simulink model "Generic_13"  (R2022b)
settings: Solver=VariableStepAuto  StartTime=0.0  StopTime=10.0  RelTol=1e-3
values from neighbouring files (symbols this model uses):
  A = cell2mat(A_cell)    [MPCController1.m]    (also in MPC_Fmincon.m)
  B = cell2mat(B_cell)    [MPCController1.m]    (also in MPC_Fmincon.m)
  brake_select = ones(length(speed), length(steering_angle))    [TwoDLook_uptable.m]
  curvature = 0.000:0.001:1    [TwoDLook_uptable.m]
  m = 1600    [MPCController1.m]    (also in MPCController2.m; MPC_Fmincon.m)
  speed = 0:0.1:100    [TwoDLook_uptable.m]
undefined symbols (not defined in the file or in its folder): Amplifier, DiscIntNeverNeededParam, K_d_yawrate, K_dsteering, k_speed, k_stanley, kd, ki, kp, path_curvature
libraries: CarMaker4SL x121, simulink x12, cstblocks x7, autolibshared x1, mpcadaslib x1
(part 2 of 5)

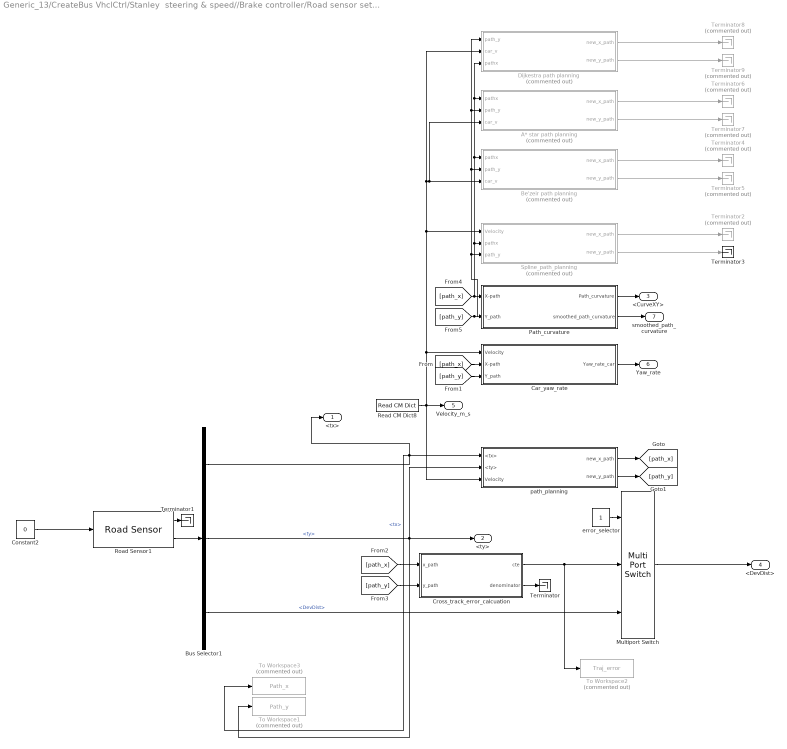
== system Generic_13/CreateBus VhclCtrl/Stanley  steering & speed//Brake controller/Road sensor set & path planning/Road sensor set & path planning ==
  A* star path planning : Subsystem  Commented=on
  Be'zeir path planning : Subsystem  Commented=on
  Bus Selector1 : BusSelector  OutputSignals=Path.tx,Path.ty,Path.DevDist
  Car_yaw_rate : Subsystem
  Constant2 : Constant  Value=0
  Cross_track_error_calcuation : Subsystem
  Dijkestra path planning : Subsystem  Commented=on
  Multiport Switch : MultiPortSwitch  Inputs=2  SaturateOnIntegerOverflow=off  InputSameDT=off
  Path_curvature : Subsystem
  Read CM Dict8 : CarMaker4SL/Read CM Dict  xname=Vhcl.v  xsync=off  xstime=Continuous
  Road Sensor1 : CarMaker4SL/Sensors/Road Sensor  xname=0  xstime=Continuous
      settings: SourceProductName=CarMaker4SL
  Spline_path_planning : Subsystem  Commented=on
  Terminator : Terminator
  Terminator1 : Terminator
  Terminator{2,4..9} (7 alike) : Terminator  Commented=on
  Terminator3 : Terminator
  To Workspace1 : ToWorkspace  Commented=on  VariableName=Path_y  SampleTime=-1
      settings: Save2DSignal=2-D array (concatenate along first dimension)
  To Workspace2 : ToWorkspace  Commented=on  VariableName=Traj_error  SampleTime=-1
      settings: Save2DSignal=2-D array (concatenate along first dimension)
  To Workspace3 : ToWorkspace  Commented=on  VariableName=Path_x  SampleTime=-1
      settings: Save2DSignal=2-D array (concatenate along first dimension)
  error_selector : Constant
  path_planning : Subsystem
  <tx> : Outport
  <ty> : Outport  Port=2
  <CurveXY> : Outport  Port=3
  <DevDist> : Outport  Port=4
  Velocity_m_s : Outport  Port=5
  Yaw_rate : Outport  Port=6
  smoothed_path_curvature : Outport  Port=7
  wires:
  [path_x] -> Car_yaw_rate/2(X-path)
  [path_x] -> Cross_track_error_calcuation/1(x_path)
  Bus Selector1/2 -> path_planning/2(<ty>), To Workspace1/1, <ty>/1  "<ty>"
  Road Sensor1/2 -> Bus Selector1/1
  Constant2/1 -> Road Sensor1/1
  Path_curvature/1(Path_curvature) -> <CurveXY>/1
  Road Sensor1/1 -> Terminator1/1
  [path_y] -> Cross_track_error_calcuation/2(y_path)
  [path_y] -> Car_yaw_rate/3(Y_path)
  Bus Selector1/1 -> path_planning/1(<tx>), To Workspace3/1, <tx>/1  "<tx>"
  Bus Selector1/3 -> Multiport Switch/3  "<DevDist>"
  error_selector/1 -> Multiport Switch/1
  Cross_track_error_calcuation/1(cte) -> To Workspace2/1, Multiport Switch/2
  Cross_track_error_calcuation/2(denominator) -> Terminator/1
  Car_yaw_rate/1(Yaw_rate_car) -> Yaw_rate/1
  path_planning/1(new_x_path) -> [path_x]
  path_planning/2(new_y_path) -> [path_y]
  Multiport Switch/1 -> <DevDist>/1
  Path_curvature/2(smoothed_path_curvature) -> smoothed_path_curvature/1
  Spline_path_planning/2(new_y_path) -> Terminator3/1
  Spline_path_planning/1(new_x_path) -> Terminator2/1
  Be'zeir path planning/1(new_x_path) -> Terminator4/1
  Be'zeir path planning/2(new_y_path) -> Terminator5/1
  [path_y] -> Dijkestra path planning/1(path_y), A* star path planning/2(path_y), Be'zeir path planning/2(path_y), Spline_path_planning/3(path_y), Path_curvature/2(Y_path)
  [path_x] -> Dijkestra path planning/3(pathx), A* star path planning/1(pathx), Be'zeir path planning/1(pathx), Spline_path_planning/2(pathx), Path_curvature/1(X-path)
  A* star path planning/2(new_y_path) -> Terminator7/1
  A* star path planning/1(new_x_path) -> Terminator6/1
  Dijkestra path planning/1(new_x_path) -> Terminator8/1
  Dijkestra path planning/2(new_y_path) -> Terminator9/1
  Read CM Dict8/1 -> Velocity_m_s/1, Dijkestra path planning/2(car_v), A* star path planning/3(car_v), Be'zeir path planning/3(car_v), Spline_path_planning/1(Velocity), Car_yaw_rate/1(Velocity), path_planning/3(Velocity)

== system Generic_13/CreateBus VhclCtrl/Stanley  steering & speed//Brake controller/Stanley controller with path_planning/Stanley controller with path_planning ==
  X-path : Inport
  Y_path : Inport  Port=2
  Discrete-Time Integrator1 : DiscreteIntegrator  Commented=on  SampleTime=-1  ICPrevOutput=DiscIntNeverNeededParam  ICPrevScaledInput=DiscIntNeverNeededParam
  MATLAB Function : MATLAB Function  Commented=on  TreatAsAtomicUnit=on
  MATLAB Function1 : MATLAB Function  Commented=on  TreatAsAtomicUnit=on
  Path_Calculation_V02 : MATLAB Function  Commented=on  TreatAsAtomicUnit=on
  Read CM Dict10 : CarMaker4SL/Read CM Dict  Commented=on  xname=Vhcl.v  xsync=off  xstime=Continuous
  Read CM Dict11 : CarMaker4SL/Read CM Dict  Commented=on  xname=Car.Gen.tx  xsync=off  xstime=Continuous
  Read CM Dict13 : CarMaker4SL/Read CM Dict  Commented=on  xname=Car.YawRate  xsync=off  xstime=Continuous
  Read CM Dict7 : CarMaker4SL/Read CM Dict  Commented=on  xname=Car.Road.Path.DevDist  xsync=off  xstime=Continuous
  Read CM Dict9 : CarMaker4SL/Read CM Dict  Commented=on  xname=Car.Gen.ty  xsync=off  xstime=Continuous
  Saturation : Saturate  Commented=on  UpperLimit=1.6  LowerLimit=-1.6
  Subsystem3 : Subsystem  Commented=on
  X_Global_Pos_m : Subsystem  Commented=on
  Y_Global_Pos_m : Subsystem  Commented=on
  Yaw_angle_rad : Subsystem  Commented=on
  e : Outport
  err_fr_axle : Outport  Port=2
  cross_track_steering : Outport  Port=3
  heading_err : Outport  Port=4
  Steering : Outport  Port=5
  closest_point : Outport  Port=6
  wires:
  X-path/1 -> Subsystem3/1(X-path)
  MATLAB Function/5(steering) -> Saturation/1
  X_Global_Pos_m/1(Pos_X) -> MATLAB Function1/1(Pos_X)
  Y_path/1 -> Subsystem3/2(Y_path)
  Subsystem3/1(x_path) -> Path_Calculation_V02/3(path_x)
  Read CM Dict13/1 -> Discrete-Time Integrator1/1, MATLAB Function/3(yaw)
  Read CM Dict9/1 -> Y_Global_Pos_m/1(In1), Path_Calculation_V02/2(y_car)
  Read CM Dict11/1 -> X_Global_Pos_m/1(In1), Path_Calculation_V02/1(x_car)
  Subsystem3/2(y_path) -> Path_Calculation_V02/4(y_path)
  Discrete-Time Integrator1/1 -> Yaw_angle_rad/1(In1)
  Y_Global_Pos_m/1(Pos_Y) -> MATLAB Function1/2(Pos_Y)
  Path_Calculation_V02/1(closest_point) -> closest_point/1
  Path_Calculation_V02/2(instantaneous_path) -> MATLAB Function1/4(Path_In)
  Yaw_angle_rad/1(Yaw_Angle) -> MATLAB Function1/3(Yaw_Angle)
  MATLAB Function1/1(Path_Out) -> MATLAB Function/1(path)
  Read CM Dict7/1 -> MATLAB Function/2(dev)
  Read CM Dict10/1 -> MATLAB Function/4(speed_act)
  MATLAB Function/1(e) -> e/1
  MATLAB Function/2(err_fr_axle) -> err_fr_axle/1
  MATLAB Function/3(cross_track_steering) -> cross_track_steering/1
  MATLAB Function/4(heading_err) -> heading_err/1
  Saturation/1 -> Steering/1  "Steering"

== system Generic_13/CreateBus VhclCtrl/Stanley  steering & speed//Brake controller/Stanley_controller_vfin/Stanley_controller_vfin ==
  Velocity : Inport
  Curvature : Inport  Port=2
  Vehicle_yaw_rate : Inport  Port=3
  Path.DevDist : Inport  Port=4
  Stanley_standfort controller : Subsystem  VariantControl=Choice
  Steering angle : Outport
  dev_angle : Outport  Port=2

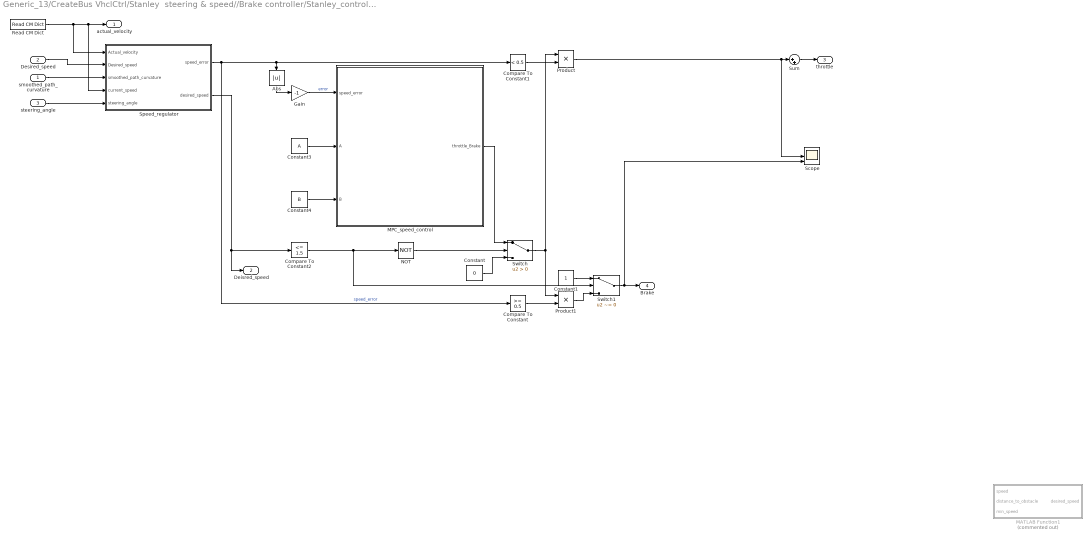
== system Generic_13/CreateBus VhclCtrl/Stanley  steering & speed//Brake controller/Stanley_controller_with_thottle_and_brake_commands/MPCLongitudianl_contorl ==
  smoothed_path_curvature : Inport
  Desired_speed : Inport  Port=2
  steering_angle : Inport  Port=3
  Abs : Abs  SaturateOnIntegerOverflow=off
  Compare To Constant : simulink/Logic and Bit Operations/Compare To Constant  relop=>=  const=0.5  OutDataTypeStr=boolean
  Compare To Constant1 : simulink/Logic and Bit Operations/Compare To Constant  relop=<  const=0.5  OutDataTypeStr=boolean
  Compare To Constant2 : simulink/Logic and Bit Operations/Compare To Constant  relop=<=  const=1.5  OutDataTypeStr=boolean
  Constant : Constant  Value=0
  Constant1 : Constant
  Constant3 : Constant  Value=A
  Constant4 : Constant  Value=B
  Gain : Gain  Gain=-1
  MATLAB Function1 : MATLAB Function  Commented=on  TreatAsAtomicUnit=on
  MPC_speed_control : MATLAB Function  TreatAsAtomicUnit=on
  NOT : Logic  Operator=NOT  IconShape=distinctive  AllPortsSameDT=off  OutDataTypeStr=boolean
  Product : Product
  Product1 : Product
  Read CM Dict : CarMaker4SL/Read CM Dict  xname=Vhcl.v  xsync=off  xstime=Continuous
  Scope : Scope  NumInputPorts=3
  Speed_regulator : Subsystem
  Sum : Sum  Inputs=|++
  Switch : Switch  Criteria=u2 > Threshold  SaturateOnIntegerOverflow=off  InputSameDT=off
  Switch1 : Switch  Criteria=u2 ~= 0  SaturateOnIntegerOverflow=off  InputSameDT=off
  actual_velocity : Outport
  Deisred_speed : Outport  Port=2
  throttle : Outport  Port=3
  Brake : Outport  Port=4
  wires:
  Read CM Dict/1 -> Speed_regulator/4(current_speed), actual_velocity/1, Speed_regulator/1(Actual_velocity)
  Abs/1 -> Gain/1
  Speed_regulator/2(desired_speed) -> Compare To Constant2/1, Deisred_speed/1
  steering_angle/1 -> Speed_regulator/5(steering_angle)
  Speed_regulator/1(speed_error) -> Compare To Constant1/1, Abs/1, Compare To Constant/1  "speed_error"
  Desired_speed/1 -> Speed_regulator/2(Desired_speed)
  smoothed_path_curvature/1 -> Speed_regulator/3(smoothed_path_curvature)
  Gain/1 -> MPC_speed_control/1(speed_error)  "error"
  Constant4/1 -> MPC_speed_control/3(B)
  Constant3/1 -> MPC_speed_control/2(A)
  Compare To Constant2/1 -> Switch1/2, NOT/1
  NOT/1 -> Switch/2
  Constant/1 -> Switch/3
  Compare To Constant1/1 -> Product/2
  Switch/1 -> Product/1, Product1/1
  Compare To Constant/1 -> Product1/2
  Product/1 -> Scope/2, Sum/1
  Constant1/1 -> Switch1/1
  Product1/1 -> Switch1/3
  Switch1/1 -> Scope/3, Brake/1
  MPC_speed_control/1(throttle_Brake) -> Switch/1
  Sum/1 -> throttle/1

== system Generic_13/CreateBus VhclCtrl/Stanley  steering & speed//Brake controller/Stanley_controller_with_thottle_and_brake_commands/Stanley steering + PID speed controller ==
  Path_out : Inport
  <Vx_Global_m_s> : Inport  Port=2
  <Vy_Global_m_s> : Inport  Port=3
  dev_angle : Inport  Port=4
  <Actual_Velocity_Car_m_s> : Inport  Port=5
  Desired_speed : Inport  Port=6
  dev_distance : Inport  Port=7
  Actual velocity [km/h] : Display
  Bus Selector : BusSelector  OutputSignals=Path.tx,Path.ty
  Constant1 : Constant  Value=0
  Delay : Delay  DelayLength=1
  Delay1 : Delay  DelayLength=1
  Gain : Gain  Gain=3.6
  Road Sensor : CarMaker4SL/Sensors/Road Sensor  xname=0  xstime=Continuous
      settings: SourceProductName=CarMaker4SL
  Saturation : Saturate  UpperLimit=pi()/2  LowerLimit=-pi/2
  Smoothing : Subsystem
  Speed_controller : Subsystem
  Stanely_controller : MATLAB Function  TreatAsAtomicUnit=on
  Subsystem1 : Subsystem
  Terminator : Terminator
  Terminator1 : Terminator
  Terminator4 : Terminator
  Steering_angle_rad : Outport  VectorParamsAs1DForOutWhenUnconnected=off
  Throttle : Outport  Port=2
  Brake_command : Outport  Port=3
  wires:
  dev_distance/1 -> Stanely_controller/2(dev)  "Dev_dis[m]"
  <Vx_Global_m_s>/1 -> Speed_controller/3(velocity_x)
  Constant1/1 -> Road Sensor/1
  dev_angle/1 -> Stanely_controller/1(dev_angle)  "dev_angle [rad]"
  <Vy_Global_m_s>/1 -> Speed_controller/4(velocity_y)
  Bus Selector/2 -> Stanely_controller/6(y2), Delay1/1  "<ty>"
  Speed_controller/4(min_safe_speed) -> Subsystem1/3(min_safe_speed)
  Road Sensor/1 -> Terminator4/1
  Road Sensor/2 -> Bus Selector/1
  Bus Selector/1 -> Stanely_controller/4(x2), Delay/1  "<tx>"
  Delay/1 -> Stanely_controller/3(x1)
  Delay1/1 -> Stanely_controller/5(y1)
  <Actual_Velocity_Car_m_s>/1 -> Speed_controller/2(speed_act), Gain/1, Stanely_controller/7(speed_act)
  Desired_speed/1 -> Subsystem1/1(desired_speed)
  Speed_controller/2(Brake_command) -> Brake_command/1
  Stanely_controller/3(steering) -> Speed_controller/6(steering), Saturation/1  "steering"
  Gain/1 -> Actual velocity [km/h]/1  "Actual velocity [km/h]"
  Path_out/1 -> Speed_controller/1(path)
  Subsystem1/1(Target_speed) -> Speed_controller/5(desired_speed)
  Saturation/1 -> Smoothing/1(Signal_In)  "Control signal"
  Speed_controller/1(Throttle) -> Throttle/1
  Speed_controller/3(path_curvature) -> Subsystem1/2(curvature)
  Smoothing/1(Signal_Out) -> Steering_angle_rad/1
  Stanely_controller/2(cross_track_steering) -> Terminator/1  "cross_track_steering"
  Stanely_controller/1(e) -> Terminator1/1  "cross track error [m]"

== system Generic_13/CreateBus VhclCtrl/Stanley  steering & speed//Brake controller/Road sensor set & path planning/Road sensor set & path planning/A* star path planning ==
  pathx : Inport
  path_y : Inport  Port=2
  car_v : Inport  Port=3
  Basic_obstacle avoidance : MATLAB Function  TreatAsAtomicUnit=on
  Demux : Demux  Commented=on
  Discrete-Time Integrator : DiscreteIntegrator  SampleTime=-1  ICPrevOutput=DiscIntNeverNeededParam  ICPrevScaledInput=DiscIntNeverNeededParam
  Mux : Mux  Inputs=2
  Mux1 : Mux  Inputs=2
  Read CM Dict : CarMaker4SL/Read CM Dict  xname=Sensor.Object.RadarL.Obj.T00.RefPnt.ds.x  xsync=off  xstime=Continuous
  Read CM Dict1 : CarMaker4SL/Read CM Dict  xname=Sensor.Object.RadarL.Obj.T00.RefPnt.ds.y  xsync=off  xstime=Continuous
  Read CM Dict2 : CarMaker4SL/Read CM Dict  xname=Car.Gen.tx  xsync=off  xstime=Continuous
  Read CM Dict3 : CarMaker4SL/Read CM Dict  xname=Car.Gen.ty  xsync=off  xstime=Continuous
  Read CM Dict4 : CarMaker4SL/Read CM Dict  xname=Sensor.Radar.VehSensor_6.Obj0.Width  xsync=off  xstime=Continuous
  Read CM Dict5 : CarMaker4SL/Read CM Dict  xname=Sensor.Radar.VehSensor_6.Obj0.Length  xsync=off  xstime=Continuous
  Read CM Dict6 : CarMaker4SL/Read CM Dict  xname=Car.YawRate  xsync=off  xstime=Continuous
  Reshape : Reshape  OutputDimensionality=Customize  OutputDimensions=[2,1]
  Reshape1 : Reshape  OutputDimensionality=Customize  OutputDimensions=[1,2]
  Reshape4 : Reshape  Commented=on
  Saturation : Saturate  UpperLimit=4  LowerLimit=-4
  Signal_smoothing : Subsystem
  Smoothing3 : Subsystem
  getInstantaneousPath Function : MATLAB Function  Commented=on  TreatAsAtomicUnit=on
  lookahead_dist : Constant  Commented=on  Value=2
  new_x_path : Outport
  new_y_path : Outport  Port=2
  wires:
  Reshape4/1 -> Demux/1
  Demux/4 -> new_y_path/1
  Basic_obstacle avoidance/1(updated_path) -> getInstantaneousPath Function/1(generated_path), Reshape4/1
  Demux/1 -> new_x_path/1
  lookahead_dist/1 -> getInstantaneousPath Function/2(lookahead_distance)
  pathx/1 -> Basic_obstacle avoidance/8(path_x), Mux1/1
  path_y/1 -> Basic_obstacle avoidance/9(path_y), Mux1/2
  car_v/1 -> Basic_obstacle avoidance/7(car_v)
  Smoothing3/1(Signal_Out) -> Basic_obstacle avoidance/5(object_length)  "steering_signal"
  Signal_smoothing/1(smoothed_width) -> Basic_obstacle avoidance/6(object_width)
  Saturation/1 -> Smoothing3/1(Signal_In)
  Discrete-Time Integrator/1 -> getInstantaneousPath Function/4(current_heading)
  Reshape/1 -> getInstantaneousPath Function/3(current_position)
  Mux1/1 -> Reshape1/1
  Read CM Dict5/1 -> Saturation/1
  Read CM Dict6/1 -> Discrete-Time Integrator/1
  Mux/1 -> Reshape/1
  Read CM Dict3/1 -> Basic_obstacle avoidance/2(Car_y), Mux/2
  Read CM Dict4/1 -> Signal_smoothing/1(Signal_In)
  Read CM Dict2/1 -> Basic_obstacle avoidance/1(Car_x), Mux/1
  Read CM Dict1/1 -> Basic_obstacle avoidance/4(dy)
  Read CM Dict/1 -> Basic_obstacle avoidance/3(dx)

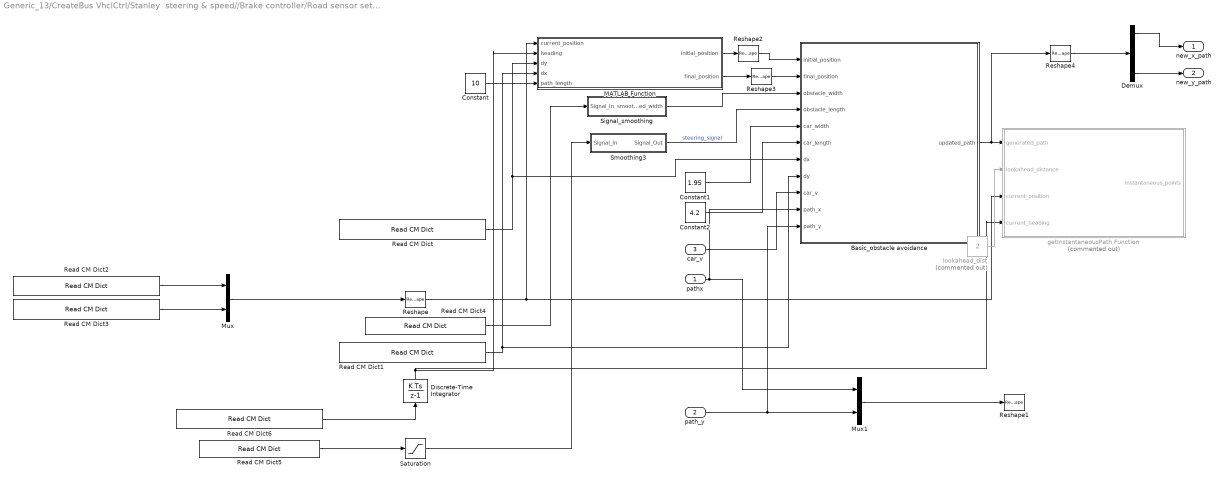
== system Generic_13/CreateBus VhclCtrl/Stanley  steering & speed//Brake controller/Road sensor set & path planning/Road sensor set & path planning/Be'zeir path planning ==
  pathx : Inport
  path_y : Inport  Port=2
  car_v : Inport  Port=3
  Basic_obstacle avoidance : MATLAB Function  TreatAsAtomicUnit=on
  Constant : Constant  Value=10
  Constant1 : Constant  Value=1.95
  Constant2 : Constant  Value=4.2
  Demux : Demux
  Discrete-Time Integrator : DiscreteIntegrator  SampleTime=-1  ICPrevOutput=DiscIntNeverNeededParam  ICPrevScaledInput=DiscIntNeverNeededParam
  MATLAB Function : MATLAB Function  TreatAsAtomicUnit=on
  Mux : Mux  Inputs=2
  Mux1 : Mux  Inputs=2
  Read CM Dict : CarMaker4SL/Read CM Dict  xname=Sensor.Object.RadarL.Obj.T00.RefPnt.ds.x  xsync=off  xstime=Continuous
  Read CM Dict1 : CarMaker4SL/Read CM Dict  xname=Sensor.Object.RadarL.Obj.T00.RefPnt.ds.y  xsync=off  xstime=Continuous
  Read CM Dict2 : CarMaker4SL/Read CM Dict  xname=Car.Gen.tx  xsync=off  xstime=Continuous
  Read CM Dict3 : CarMaker4SL/Read CM Dict  xname=Car.Gen.ty  xsync=off  xstime=Continuous
  Read CM Dict4 : CarMaker4SL/Read CM Dict  xname=Sensor.Radar.VehSensor_6.Obj0.Width  xsync=off  xstime=Continuous
  Read CM Dict5 : CarMaker4SL/Read CM Dict  xname=Sensor.Radar.VehSensor_6.Obj0.Length  xsync=off  xstime=Continuous
  Read CM Dict6 : CarMaker4SL/Read CM Dict  xname=Car.YawRate  xsync=off  xstime=Continuous
  Reshape : Reshape  OutputDimensionality=Customize  OutputDimensions=[2,1]
  Reshape1 : Reshape  OutputDimensionality=Customize  OutputDimensions=[1,2]
  Reshape2 : Reshape  OutputDimensionality=Customize  OutputDimensions=[1,2]
  Reshape3 : Reshape  OutputDimensionality=Customize  OutputDimensions=[1,2]
  Reshape4 : Reshape
  Saturation : Saturate  UpperLimit=4  LowerLimit=-4
  Signal_smoothing : Subsystem
  Smoothing3 : Subsystem
  getInstantaneousPath Function : MATLAB Function  Commented=on  TreatAsAtomicUnit=on
  lookahead_dist : Constant  Commented=on  Value=2
  new_x_path : Outport
  new_y_path : Outport  Port=2
  wires:
  Read CM Dict1/1 -> Basic_obstacle avoidance/8(dy), MATLAB Function/4(dx)
  Read CM Dict2/1 -> Mux/1
  MATLAB Function/2(final_position) -> Reshape3/1
  Constant/1 -> MATLAB Function/5(path_length)
  Read CM Dict4/1 -> Signal_smoothing/1(Signal_In)
  Read CM Dict3/1 -> Mux/2
  Mux/1 -> Reshape/1
  Read CM Dict6/1 -> Discrete-Time Integrator/1
  Read CM Dict5/1 -> Saturation/1
  Mux1/1 -> Reshape1/1
  Read CM Dict/1 -> Basic_obstacle avoidance/7(dx), MATLAB Function/3(dy)
  Reshape/1 -> getInstantaneousPath Function/3(current_position), MATLAB Function/1(current_position)
  Discrete-Time Integrator/1 -> MATLAB Function/2(heading), getInstantaneousPath Function/4(current_heading)
  Saturation/1 -> Smoothing3/1(Signal_In)
  MATLAB Function/1(initial_position) -> Reshape2/1
  Signal_smoothing/1(smoothed_width) -> Basic_obstacle avoidance/3(obstacle_width)
  Constant1/1 -> Basic_obstacle avoidance/5(car_width)
  Smoothing3/1(Signal_Out) -> Basic_obstacle avoidance/4(obstacle_length)  "steering_signal"
  Constant2/1 -> Basic_obstacle avoidance/6(car_length)
  car_v/1 -> Basic_obstacle avoidance/9(car_v)
  path_y/1 -> Mux1/2, Basic_obstacle avoidance/11(path_y)
  pathx/1 -> Mux1/1, Basic_obstacle avoidance/10(path_x)
  lookahead_dist/1 -> getInstantaneousPath Function/2(lookahead_distance)
  Reshape2/1 -> Basic_obstacle avoidance/1(initial_position)
  Reshape3/1 -> Basic_obstacle avoidance/2(final_position)
  Demux/1 -> new_x_path/1
  Basic_obstacle avoidance/1(updated_path) -> Reshape4/1, getInstantaneousPath Function/1(generated_path)
  Demux/4 -> new_y_path/1
  Reshape4/1 -> Demux/1

== system Generic_13/CreateBus VhclCtrl/Stanley  steering & speed//Brake controller/Road sensor set & path planning/Road sensor set & path planning/Car_yaw_rate ==
  Velocity : Inport
  X-path : Inport  Port=2
  Y_path : Inport  Port=3
  " Path_expanding1" : Subsystem
  Constant : Constant  Value=20
  Gain2 : Gain  Gain=-1
  Multiport Switch : MultiPortSwitch  Inputs=2  SaturateOnIntegerOverflow=off  InputSameDT=off
  Multiport Switch1 : MultiPortSwitch  Inputs=2  SaturateOnIntegerOverflow=off  InputSameDT=off
  Product3 : Product
  Read CM Dict5 : CarMaker4SL/Read CM Dict  xname=Car.YawRate  xsync=off  xstime=Continuous
  Saturation3 : Saturate  UpperLimit=5  LowerLimit=-5
  Varying Lowpass Filter1 : cstblocks/Linear Parameter Varying/Varying Lowpass Filter  N=1
  Vehicle_yaw_rate_selcotr : Constant
  Yaw_rate_filter_slector : Constant
  calculate_path_curvature2 : MATLAB Function  TreatAsAtomicUnit=on  VariantControl=Choice
  Yaw_rate_car : Outport
  wires:
  " Path_expanding1"/1(x_path) -> calculate_path_curvature2/1(path_x)
  X-path/1 -> " Path_expanding1"/1(X-path)
  Gain2/1 -> Multiport Switch1/2, Saturation3/1
  Y_path/1 -> " Path_expanding1"/2(Y_path)
  Velocity/1 -> Product3/1
  " Path_expanding1"/2(y_path) -> calculate_path_curvature2/2(path_y)
  Product3/1 -> Gain2/1
  calculate_path_curvature2/1(path_curvature) -> Product3/2
  Saturation3/1 -> Varying Lowpass Filter1/1
  Constant/1 -> Varying Lowpass Filter1/2
  Yaw_rate_filter_slector/1 -> Multiport Switch1/1
  Varying Lowpass Filter1/1 -> Multiport Switch1/3  "Yaw_rate_car"
  Vehicle_yaw_rate_selcotr/1 -> Multiport Switch/1
  Multiport Switch1/1 -> Multiport Switch/2
  Read CM Dict5/1 -> Multiport Switch/3
  Multiport Switch/1 -> Yaw_rate_car/1  "Yaw_rate_car"

== system Generic_13/CreateBus VhclCtrl/Stanley  steering & speed//Brake controller/Road sensor set & path planning/Road sensor set & path planning/Cross_track_error_calcuation ==
  x_path : Inport
  y_path : Inport  Port=2
  Constant : Constant  Value=25
  Cross_track_error_calcuation : MATLAB Function  TreatAsAtomicUnit=on
  Delay : Delay  DelayLength=1  InitialCondition=0.1
  Delay1 : Delay  DelayLength=1  InitialCondition=0.1
  Gain1 : Gain  Gain=-1
  Read CM Dict12 : CarMaker4SL/Read CM Dict  xname=Car.Gen.ty  xsync=off  xstime=Continuous
  Read CM Dict8 : CarMaker4SL/Read CM Dict  xname=Car.Gen.tx  xsync=off  xstime=Continuous
  Saturation1 : Saturate  UpperLimit=7  LowerLimit=-7
  Varying Lowpass Filter2 : cstblocks/Linear Parameter Varying/Varying Lowpass Filter  N=1
  cte : Outport
  denominator : Outport  Port=2
  wires:
  Read CM Dict12/1 -> Cross_track_error_calcuation/2(y_vehicle)
  x_path/1 -> Cross_track_error_calcuation/5(x2), Delay1/1
  Saturation1/1 -> Varying Lowpass Filter2/1
  Delay/1 -> Cross_track_error_calcuation/4(y_point)
  Cross_track_error_calcuation/2(denominator) -> denominator/1
  y_path/1 -> Cross_track_error_calcuation/6(y2), Delay/1
  Delay1/1 -> Cross_track_error_calcuation/3(x_point)
  Read CM Dict8/1 -> Cross_track_error_calcuation/1(x_vehicle)
  Cross_track_error_calcuation/1(cte) -> Gain1/1
  Gain1/1 -> Saturation1/1
  Constant/1 -> Varying Lowpass Filter2/2
  Varying Lowpass Filter2/1 -> cte/1

== system Generic_13/CreateBus VhclCtrl/Stanley  steering & speed//Brake controller/Road sensor set & path planning/Road sensor set & path planning/Dijkestra path planning ==
  path_y : Inport
  car_v : Inport  Port=2
  pathx : Inport  Port=3
  Basic_obstacle avoidance : MATLAB Function  TreatAsAtomicUnit=on
  Demux : Demux  Commented=on
  Discrete-Time Integrator : DiscreteIntegrator  SampleTime=-1  ICPrevOutput=DiscIntNeverNeededParam  ICPrevScaledInput=DiscIntNeverNeededParam
  Mux : Mux  Inputs=2
  Mux1 : Mux  Inputs=2
  Read CM Dict : CarMaker4SL/Read CM Dict  xname=Sensor.Object.RadarL.Obj.T00.RefPnt.ds.x  xsync=off  xstime=Continuous
  Read CM Dict1 : CarMaker4SL/Read CM Dict  xname=Sensor.Object.RadarL.Obj.T00.RefPnt.ds.y  xsync=off  xstime=Continuous
  Read CM Dict2 : CarMaker4SL/Read CM Dict  xname=Car.Gen.tx  xsync=off  xstime=Continuous
  Read CM Dict3 : CarMaker4SL/Read CM Dict  xname=Car.Gen.ty  xsync=off  xstime=Continuous
  Read CM Dict4 : CarMaker4SL/Read CM Dict  xname=Sensor.Radar.VehSensor_6.Obj0.Width  xsync=off  xstime=Continuous
  Read CM Dict5 : CarMaker4SL/Read CM Dict  xname=Sensor.Radar.VehSensor_6.Obj0.Length  xsync=off  xstime=Continuous
  Read CM Dict6 : CarMaker4SL/Read CM Dict  xname=Car.YawRate  xsync=off  xstime=Continuous
  Reshape : Reshape  OutputDimensionality=Customize  OutputDimensions=[2,1]
  Reshape1 : Reshape  OutputDimensionality=Customize  OutputDimensions=[1,2]
  Reshape4 : Reshape  Commented=on
  Saturation : Saturate  UpperLimit=4  LowerLimit=-4
  Signal_smoothing : Subsystem
  Smoothing3 : Subsystem
  getInstantaneousPath Function : MATLAB Function  Commented=on  TreatAsAtomicUnit=on
  lookahead_dist : Constant  Commented=on  Value=2
  new_x_path : Outport
  new_y_path : Outport  Port=2
  wires:
  Read CM Dict/1 -> Basic_obstacle avoidance/3(dx)
  Read CM Dict1/1 -> Basic_obstacle avoidance/4(dy)
  Read CM Dict2/1 -> Mux/1, Basic_obstacle avoidance/1(Car_x)
  Read CM Dict4/1 -> Signal_smoothing/1(Signal_In)
  Read CM Dict3/1 -> Mux/2, Basic_obstacle avoidance/2(Car_y)
  Mux/1 -> Reshape/1
  Read CM Dict6/1 -> Discrete-Time Integrator/1
  Read CM Dict5/1 -> Saturation/1
  Mux1/1 -> Reshape1/1
  Reshape/1 -> getInstantaneousPath Function/3(current_position)
  Discrete-Time Integrator/1 -> getInstantaneousPath Function/4(current_heading)
  Saturation/1 -> Smoothing3/1(Signal_In)
  Signal_smoothing/1(smoothed_width) -> Basic_obstacle avoidance/6(object_width)
  Smoothing3/1(Signal_Out) -> Basic_obstacle avoidance/5(object_length)  "steering_signal"
  car_v/1 -> Basic_obstacle avoidance/7(car_v)
  path_y/1 -> Mux1/2, Basic_obstacle avoidance/9(path_y)
  pathx/1 -> Mux1/1, Basic_obstacle avoidance/8(path_x)
  lookahead_dist/1 -> getInstantaneousPath Function/2(lookahead_distance)
  Demux/1 -> new_x_path/1
  Basic_obstacle avoidance/1(updated_path) -> Reshape4/1, getInstantaneousPath Function/1(generated_path)
  Demux/4 -> new_y_path/1
  Reshape4/1 -> Demux/1

== system Generic_13/CreateBus VhclCtrl/Stanley  steering & speed//Brake controller/Road sensor set & path planning/Road sensor set & path planning/Path_curvature ==
  X-path : Inport
  Y_path : Inport  Port=2
  " Path_expanding" : Subsystem
  Constant : Constant  Value=25
  Multiport Switch : MultiPortSwitch  Inputs=2  SaturateOnIntegerOverflow=off  InputSameDT=off
  Multiport Switch1 : MultiPortSwitch  Inputs=2  SaturateOnIntegerOverflow=off  InputSameDT=off
  Read CM Dict6 : CarMaker4SL/Read CM Dict  xname=Sensor.Road.VehSensor_0.Path.CurveXY  xsync=off  xstime=Continuous
  Saturation2 : Saturate  UpperLimit=1  LowerLimit=-1
  Scope : Scope
  Varying Lowpass Filter : cstblocks/Linear Parameter Varying/Varying Lowpass Filter  N=1
  calculate_path_curvature1 : MATLAB Function  TreatAsAtomicUnit=on  VariantControl=Choice
  inverting : Gain  Gain=-1
  path_curv_selector : Constant
  path_curv_selector1 : Constant
  Path_curvature : Outport
  smoothed_path_curvature : Outport  Port=2
  wires:
  inverting/1 -> Multiport Switch1/2, Saturation2/1
  X-path/1 -> " Path_expanding"/1(X-path)
  Y_path/1 -> " Path_expanding"/2(Y_path)
  " Path_expanding"/1(x_path) -> calculate_path_curvature1/1(path_x)
  calculate_path_curvature1/1(path_curvature) -> inverting/1
  Read CM Dict6/1 -> Multiport Switch/3
  " Path_expanding"/2(y_path) -> calculate_path_curvature1/2(path_y)
  Saturation2/1 -> Varying Lowpass Filter/1
  Varying Lowpass Filter/1 -> Scope/1, smoothed_path_curvature/1, Multiport Switch1/3  "Path_curvature"
  Constant/1 -> Varying Lowpass Filter/2
  path_curv_selector1/1 -> Multiport Switch1/1
  path_curv_selector/1 -> Multiport Switch/1
  Multiport Switch1/1 -> Multiport Switch/2
  Multiport Switch/1 -> Path_curvature/1  "Path_curvature"

== system Generic_13/CreateBus VhclCtrl/Stanley  steering & speed//Brake controller/Road sensor set & path planning/Road sensor set & path planning/Spline_path_planning ==
  Velocity : Inport
  pathx : Inport  Port=2
  path_y : Inport  Port=3
  Demux : Demux  Outputs=2
  Discrete-Time Integrator : DiscreteIntegrator  SampleTime=-1  ICPrevOutput=DiscIntNeverNeededParam  ICPrevScaledInput=DiscIntNeverNeededParam
  Mux : Mux  Inputs=2
  Mux1 : Mux  Inputs=2
  Read CM Dict : CarMaker4SL/Read CM Dict  xname=Sensor.Object.RadarL.Obj.T00.RefPnt.ds.x  xsync=off  xstime=Continuous
  Read CM Dict1 : CarMaker4SL/Read CM Dict  xname=Sensor.Object.RadarL.Obj.T00.RefPnt.ds.y  xsync=off  xstime=Continuous
  Read CM Dict2 : CarMaker4SL/Read CM Dict  xname=Car.Gen.tx  xsync=off  xstime=Continuous
  Read CM Dict3 : CarMaker4SL/Read CM Dict  xname=Car.Gen.ty  xsync=off  xstime=Continuous
  Read CM Dict4 : CarMaker4SL/Read CM Dict  xname=Sensor.Radar.VehSensor_6.Obj0.Width  xsync=off  xstime=Continuous
  Read CM Dict5 : CarMaker4SL/Read CM Dict  xname=Sensor.Radar.VehSensor_6.Obj0.Length  xsync=off  xstime=Continuous
  Read CM Dict6 : CarMaker4SL/Read CM Dict  xname=Car.YawRate  xsync=off  xstime=Continuous
  Reshape : Reshape  OutputDimensionality=Customize  OutputDimensions=[1,2]
  Reshape1 : Reshape  OutputDimensionality=Customize  OutputDimensions=[1,2]
  Saturation : Saturate  UpperLimit=4  LowerLimit=-4
  Signal_smoothing : Subsystem
  Smoothing3 : Subsystem
  Spline_bsed_obstacle avoidance : MATLAB Function  TreatAsAtomicUnit=on
  getInstantaneousPath Function : MATLAB Function  TreatAsAtomicUnit=on
  lookahead_dist : Constant  Value=2
  new_x_path : Outport
  new_y_path : Outport  Port=2
  wires:
  Signal_smoothing/1(smoothed_width) -> Spline_bsed_obstacle avoidance/5(object_width)
  Read CM Dict4/1 -> Signal_smoothing/1(Signal_In)
  Demux/1 -> new_x_path/1
  Demux/2 -> new_y_path/1
  Spline_bsed_obstacle avoidance/1(updated_path) -> getInstantaneousPath Function/1(generated_path)  "generated_path"
  Smoothing3/1(Signal_Out) -> Spline_bsed_obstacle avoidance/6(object_length)  "steering_signal"
  Read CM Dict1/1 -> Spline_bsed_obstacle avoidance/4(dy)
  Read CM Dict/1 -> Spline_bsed_obstacle avoidance/3(dx)
  Saturation/1 -> Smoothing3/1(Signal_In)
  Velocity/1 -> Spline_bsed_obstacle avoidance/7(car_v)
  Read CM Dict5/1 -> Saturation/1
  Read CM Dict3/1 -> Mux/2, Spline_bsed_obstacle avoidance/2(Car_y)  "car_y"
  Read CM Dict2/1 -> Mux/1, Spline_bsed_obstacle avoidance/1(Car_x)  "car_x"
  Mux/1 -> Reshape/1
  Reshape/1 -> getInstantaneousPath Function/3(current_position)
  lookahead_dist/1 -> getInstantaneousPath Function/2(lookahead_distance)
  Read CM Dict6/1 -> Discrete-Time Integrator/1
  Discrete-Time Integrator/1 -> getInstantaneousPath Function/4(current_heading)
  Mux1/1 -> Reshape1/1
  pathx/1 -> Spline_bsed_obstacle avoidance/8(pathx), Mux1/1
  path_y/1 -> Spline_bsed_obstacle avoidance/9(path_y), Mux1/2
  getInstantaneousPath Function/1(instantaneous_points) -> Demux/1

== system Generic_13/CreateBus VhclCtrl/Stanley  steering & speed//Brake controller/Road sensor set & path planning/Road sensor set & path planning/path_planning ==
  <tx> : Inport
  <ty> : Inport  Port=2
  Velocity : Inport  Port=3
  Basic_obstacle avoidance : MATLAB Function  TreatAsAtomicUnit=on
  Demux : Demux  Outputs=2
  Floor : Rounding  Operator=ceil
  Read CM Dict : CarMaker4SL/Read CM Dict  xname=Sensor.Object.FrontRadar.Obj.T00.RefPnt.ds.x  xsync=off  xstime=Continuous
  Read CM Dict1 : CarMaker4SL/Read CM Dict  xname=Sensor.Object.FrontRadar.Obj.T00.RefPnt.ds.y  xsync=off  xstime=Continuous
  Read CM Dict2 : CarMaker4SL/Read CM Dict  xname=Car.Gen.tx  xsync=off  xstime=Continuous
  Read CM Dict3 : CarMaker4SL/Read CM Dict  xname=Car.Gen.ty  xsync=off  xstime=Continuous
  Read CM Dict4 : CarMaker4SL/Read CM Dict  xname=Sensor.Radar.VehSensor_6.Obj0.Width  xsync=off  xstime=Continuous
  Read CM Dict5 : CarMaker4SL/Read CM Dict  xname=Sensor.Radar.VehSensor_6.Obj0.Length  xsync=off  xstime=Continuous
  Saturation : Saturate  UpperLimit=4  LowerLimit=-4
  Signal_smoothing : Subsystem
  Smoothing3 : Subsystem
  To Workspace1 : ToWorkspace  VariableName=CarY  SampleTime=-1
      settings: Save2DSignal=2-D array (concatenate along first dimension)
  To Workspace3 : ToWorkspace  VariableName=CarX  SampleTime=-1
      settings: Save2DSignal=2-D array (concatenate along first dimension)
  new_x_path : Outport
  new_y_path : Outport  Port=2
  wires:
  Read CM Dict2/1 -> To Workspace3/1, Basic_obstacle avoidance/1(Car_x)
  Read CM Dict3/1 -> To Workspace1/1, Basic_obstacle avoidance/2(Car_y)
  Read CM Dict5/1 -> Saturation/1
  Velocity/1 -> Basic_obstacle avoidance/9(car_v), Floor/1
  Saturation/1 -> Smoothing3/1(Signal_In)
  Read CM Dict/1 -> Basic_obstacle avoidance/3(dx)
  Read CM Dict1/1 -> Basic_obstacle avoidance/4(dy)
  Smoothing3/1(Signal_Out) -> Basic_obstacle avoidance/6(object_length)  "steering_signal"
  <tx>/1 -> Basic_obstacle avoidance/7(path_x)
  <ty>/1 -> Basic_obstacle avoidance/8(path_y)
  Floor/1 -> Basic_obstacle avoidance/10(car_v_ceil)
  Basic_obstacle avoidance/1(updated_path) -> Demux/1
  Demux/2 -> new_y_path/1
  Demux/1 -> new_x_path/1
  Read CM Dict4/1 -> Signal_smoothing/1(Signal_In)
  Signal_smoothing/1(smoothed_width) -> Basic_obstacle avoidance/5(object_width)

== system Generic_13/CreateBus VhclCtrl/Stanley  steering & speed//Brake controller/Stanley controller with path_planning/Stanley controller with path_planning/Subsystem3 ==
  X-path : Inport
  Y_path : Inport  Port=2
  Delay37 : Delay  DelayLength=1
  Delay4 : Delay  DelayLength=1
  Mux1 : Mux  Inputs=2
  Mux2 : Mux  Inputs=2
  Reshape1 : Reshape  OutputDimensionality=Customize  OutputDimensions=[1,2]
  Reshape2 : Reshape  OutputDimensionality=Customize  OutputDimensions=[1,2]
  x_path : Outport
  y_path : Outport  Port=2
  wires:
  X-path/1 -> Delay37/1, Mux2/1
  Y_path/1 -> Delay4/1, Mux1/1
  Delay37/1 -> Mux2/2
  Mux1/1 -> Reshape1/1
  Reshape1/1 -> y_path/1
  Delay4/1 -> Mux1/2
  Reshape2/1 -> x_path/1
  Mux2/1 -> Reshape2/1

== system Generic_13/CreateBus VhclCtrl/Stanley  steering & speed//Brake controller/Stanley controller with path_planning/Stanley controller with path_planning/X_Global_Pos_m ==
  In1 : Inport
  Pos_X : Outport  VectorParamsAs1DForOutWhenUnconnected=off
  wires:
  In1/1 -> Pos_X/1

== system Generic_13/CreateBus VhclCtrl/Stanley  steering & speed//Brake controller/Stanley controller with path_planning/Stanley controller with path_planning/Y_Global_Pos_m ==
  In1 : Inport
  Pos_Y : Outport  VectorParamsAs1DForOutWhenUnconnected=off
  wires:
  In1/1 -> Pos_Y/1

== system Generic_13/CreateBus VhclCtrl/Stanley  steering & speed//Brake controller/Stanley controller with path_planning/Stanley controller with path_planning/Yaw_angle_rad ==
  In1 : Inport
  Yaw_Angle : Outport  VectorParamsAs1DForOutWhenUnconnected=off
  wires:
  In1/1 -> Yaw_Angle/1

== system Generic_13/CreateBus VhclCtrl/Stanley  steering & speed//Brake controller/Stanley_controller_vfin/Stanley_controller_vfin/Stanley_standfort controller ==
  note: Vehicle_paramters
  note: Parameters
  note: K_dsteering = 10;
  note: Amplifier = -5.94
  note: K_d_yawrate =0.4
  note: Vehicle overall mass [kg] 	: 	1600.00
      |
      |  Vehicle overall center of gravity x / y / z [m] 	: 	2.596	0.000	0.562
      |
      |  Vehicle overall inertia tensor [kgm²] 	: 	696.215	0.000	-8.863
      |  	 									0.000	2707.206	0.000
      |  	 									-8.863	0.000	2986.624
  note: Distance CoG to front axle / rear axle [m] : 1.488 -1.487
  note: k_stanly = 13.6;
  Velocity : Inport
  Curvature : Inport  Port=2
  Vehicle_yaw_rate : Inport  Port=3
  Path.DevDist : Inport  Port=4
  Add : Sum  Inputs=+++
  Add1 : Sum
  Crosstrack_steering : Subsystem
  Deviation_angle_calc : Subsystem
  Scope : Scope  NumInputPorts=2
  Steady_state_yaw : Subsystem  Commented=on
  Steering_correction_facotr : Subsystem
  Yaw_rate_diff : Subsystem
  Steering angle : Outport
  dev_angle : Outport  Port=2
  wires:
  Velocity/1 -> Crosstrack_steering/1(speed), Deviation_angle_calc/1(Velocity), Yaw_rate_diff/1(Velocity)
  Crosstrack_steering/1(Cross_track_steering) -> Add/1  "Crosstrack_steering"
  Add/1 -> Add1/1
  Add1/1 -> Steering angle/1, Steering_correction_facotr/1(Steering_i+1), Steering_correction_facotr/2(Steering_i)  "Steering angle"
  Deviation_angle_calc/1(Dev_angle) -> dev_angle/1, Add/3
  Steering_correction_facotr/1(Factor_of_correction) -> Add1/2
  Yaw_rate_diff/1(Yaw_rate_factor) -> Add/2
  Vehicle_yaw_rate/1 -> Yaw_rate_diff/3(Car_yaw_rate), Deviation_angle_calc/3(Car.YawRate), Scope/2
  Path.DevDist/1 -> Crosstrack_steering/2(Path.DevDist)
  Curvature/1 -> Scope/1, Deviation_angle_calc/2(Curvature), Yaw_rate_diff/2(Curvature)

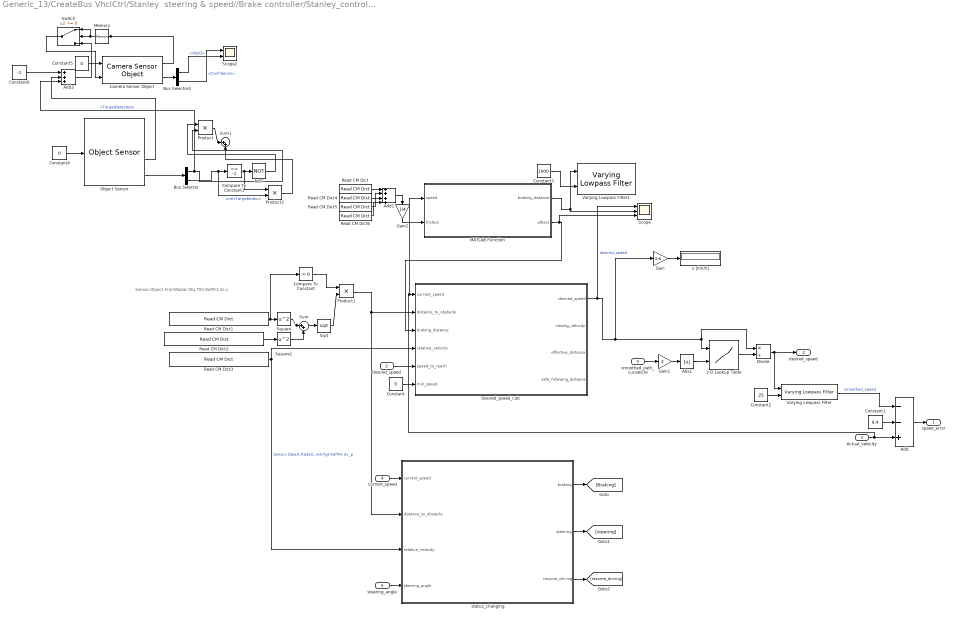
== system Generic_13/CreateBus VhclCtrl/Stanley  steering & speed//Brake controller/Stanley_controller_with_thottle_and_brake_commands/MPCLongitudianl_contorl/Speed_regulator ==
  note: Sensor.Object.FrontRadar.Obj.T00.RefPnt.ds.x
  Actual_velocity : Inport
  Desired_speed : Inport  Port=2
  smoothed_path_curvature : Inport  Port=3
  current_speed : Inport  Port=4
  steering_angle : Inport  Port=5
  2-D Lookup Table : Lookup_n-D  BreakpointsForDimension1=speed  BreakpointsForDimension2=curvature  Table=brake_select  InternalRulePriority=Speed  RndMeth=Simplest
      settings: InputPortMap=u0,u1
  Abs2 : Abs  SaturateOnIntegerOverflow=off
  Add : Sum  Inputs=--+
  Add1 : Sum  Inputs=++++
  Add2 : Sum  Inputs=+++
  Bus Selector : BusSelector  OutputSignals=TargetDetected,relvTargetIndex
  Bus Selector4 : BusSelector  OutputSignals=ObjID,Confidence
  Camera Sensor Object : CarMaker4SL/Sensors/Camera Sensor Object  xname=INPORT  xstime=Continuous
      settings: SourceProductName=CarMaker4SL
  Compare To Constant : simulink/Logic and Bit Operations/Compare To Constant  relop=>  const=0  OutDataTypeStr=boolean
  Compare To Constant1 : simulink/Logic and Bit Operations/Compare To Constant  relop===  const=-1  OutDataTypeStr=boolean
  Constant : Constant  Value=0
  Constant1 : Constant  Value=0.4
  Constant2 : Constant  Value=25
  Constant3 : Constant  Value=1000
  Constant4 : Constant  Value=0
  Constant5 : Constant  Value=0
  Constant6 : Constant  Value=-1
  Desired_speed_calc : MATLAB Function  TreatAsAtomicUnit=on
  Divide : Product  Inputs=*/
  Gain : Gain  Gain=3.6
  Gain1 : Gain  Gain=2
  Gain2 : Gain  Gain=1/4
  MATLAB Function : MATLAB Function  TreatAsAtomicUnit=on
  Memory : Memory
  NOT : Logic  Operator=NOT  IconShape=distinctive  AllPortsSameDT=off  OutDataTypeStr=boolean
  Object Sensor : CarMaker4SL/Sensors/Object Sensor  xname=INPORT  xstime=Continuous
      settings: SourceProductName=CarMaker4SL
  Product : Product
  Product1 : Product
  Product2 : Product
  Read CM Dict : CarMaker4SL/Read CM Dict  xname=Car.muRoadFL  xsync=off  xstime=Continuous
  Read CM Dict1 : CarMaker4SL/Read CM Dict  xname=Sensor.Object.FrontRadar.Obj.T01.RefPnt.ds.x  xsync=off  xstime=Continuous
  Read CM Dict2 : CarMaker4SL/Read CM Dict  xname=Sensor.Object.FrontRadar.Obj.T01.RefPnt.ds.y  xsync=off  xstime=Continuous
  Read CM Dict3 : CarMaker4SL/Read CM Dict  xname=Sensor.Object.FrontRadar.relvTgt.RefPnt.dv_p  xsync=off  xstime=Continuous
  Read CM Dict4 : CarMaker4SL/Read CM Dict  xname=Car.muRoadFR  xsync=off  xstime=Continuous
  Read CM Dict5 : CarMaker4SL/Read CM Dict  xname=Car.muRoadRL  xsync=off  xstime=Continuous
  Read CM Dict6 : CarMaker4SL/Read CM Dict  xname=Car.muRoadRR  xsync=off  xstime=Continuous
  Scope : Scope  NumInputPorts=3
  Scope2 : Scope  NumInputPorts=2
  Sqrt : Sqrt
  Square : Math  Operator=square
  Square1 : Math  Operator=square
  Sum : Sum  Inputs=|++
  Sum1 : Sum  Inputs=|++
  Switch : Switch  SaturateOnIntegerOverflow=off  InputSameDT=off
  Varying Lowpass Filter : cstblocks/Linear Parameter Varying/Varying Lowpass Filter  N=1
  Varying Lowpass Filter1 : cstblocks/Linear Parameter Varying/Varying Lowpass Filter  N=1
  status_changing : MATLAB Function  TreatAsAtomicUnit=on
  v [km/h] : Display
  speed_error : Outport
  desired_speed : Outport  Port=2
  wires:
  Gain1/1 -> Abs2/1
  Constant/1 -> Desired_speed_calc/6(min_speed)
  Sqrt/1 -> Product1/2
  Desired_speed/1 -> Desired_speed_calc/5(speed_to_reach)
  Abs2/1 -> 2-D Lookup Table/2
  Read CM Dict3/1 -> status_changing/3(relative_velocity), Desired_speed_calc/4(relative_velocity)  "Sensor.Object.RadarL.relvTgt.RefPnt.dv_p"
  Constant1/1 -> Add/2
  Product1/1 -> status_changing/2(distance_to_obstacle), Desired_speed_calc/2(distance_to_obstacle)
  Desired_speed_calc/1(desired_speed) -> Scope/1, Gain/1, Divide/1, 2-D Lookup Table/1  "desired_speed"
  Read CM Dict2/1 -> Square1/1
  steering_angle/1 -> status_changing/4(steering_angle)
  Square1/1 -> Sum/2
  Gain/1 -> v [km/h]/1
  2-D Lookup Table/1 -> Divide/2
  status_changing/3(resume_driving) -> [resume_driving]
  Sum/1 -> Sqrt/1
  Square/1 -> Sum/1
  Add/1 -> speed_error/1
  smoothed_path_curvature/1 -> Gain1/1
  Compare To Constant/1 -> Product1/1
  Read CM Dict1/1 -> Compare To Constant/1, Square/1
  status_changing/2(steering) -> [steering]
  status_changing/1(braking) -> [Braking]
  current_speed/1 -> status_changing/1(current_speed)
  Constant2/1 -> Varying Lowpass Filter/2
  Divide/1 -> desired_speed/1, Varying Lowpass Filter/1
  Varying Lowpass Filter/1 -> Add/1  "smoothed_speed"
  Actual_velocity/1 -> MATLAB Function/1(speed), Desired_speed_calc/1(current_speed), Add/3
  MATLAB Function/1(braking_distance) -> Varying Lowpass Filter1/1, Scope/2
  Constant3/1 -> Varying Lowpass Filter1/2
  Read CM Dict/1 -> Add1/1
  Read CM Dict4/1 -> Add1/2
  Read CM Dict5/1 -> Add1/3
  Read CM Dict6/1 -> Add1/4
  Add1/1 -> Gain2/1
  MATLAB Function/2(others) -> Scope/3, Desired_speed_calc/3(braking_distance)
  Gain2/1 -> MATLAB Function/2(friction)
  Object Sensor/3 -> Add2/2
  Constant4/1 -> Object Sensor/1
  Object Sensor/4 -> Bus Selector/1
  Bus Selector/2 -> Product2/2, Compare To Constant1/1  "<relvTargetIndex>"
  Compare To Constant1/1 -> Product2/1, NOT/1
  NOT/1 -> Product/1
  Product2/1 -> Sum1/2
  Bus Selector/1 -> Add2/3, Product/2  "<TargetDetected>"
  Product/1 -> Sum1/1
  Camera Sensor Object/2 -> Bus Selector4/1
  Bus Selector4/1 -> Scope2/2  "<ObjID>"
  Constant5/1 -> Camera Sensor Object/1
  Bus Selector4/2 -> Scope2/1  "<Confidence>"
  Add2/1 -> Switch/3
  Constant6/1 -> Add2/1
  Camera Sensor Object/1 -> Memory/1
  Switch/1 -> Camera Sensor Object/2
  Memory/1 -> Switch/1, Switch/2

== system Generic_13/CreateBus VhclCtrl/Stanley  steering & speed//Brake controller/Stanley_controller_with_thottle_and_brake_commands/Stanley steering + PID speed controller/Smoothing ==
  Signal_In : Inport
  Add : Sum  Inputs=++++
  Delay : Delay  InitialCondition=0.1
  Delay1 : Delay  DelayLength=4  InitialCondition=0.1
  Delay2 : Delay  DelayLength=5  InitialCondition=0.1
  Gain : Gain  Gain=0.35
  Gain1 : Gain  Gain=0.25
  Gain2 : Gain  Gain=0.25
  Gain3 : Gain  Gain=0.15
  Signal_Out : Outport  VectorParamsAs1DForOutWhenUnconnected=off
  wires:
  Gain1/1 -> Add/2
  Signal_In/1 -> Gain/1
  Delay/1 -> Gain1/1
  Gain/1 -> Add/1
  Delay1/1 -> Gain2/1
  Add/1 -> Delay2/1, Delay1/1, Delay/1, Signal_Out/1
  Gain2/1 -> Add/3
  Delay2/1 -> Gain3/1
  Gain3/1 -> Add/4

== system Generic_13/CreateBus VhclCtrl/Stanley  steering & speed//Brake controller/Stanley_controller_with_thottle_and_brake_commands/Stanley steering + PID speed controller/Speed_controller ==
  path : Inport
  speed_act : Inport  Port=2
  velocity_x : Inport  Port=3
  velocity_y : Inport  Port=4
  desired_speed : Inport  Port=5
  steering : Inport  Port=6
  Brake Saturation : Saturate  UpperLimit=1  LowerLimit=0
  Constant1 : Constant  Value=kd
  Constant2 : Constant  Value=ki
  Constant3 : Constant  Value=kp
  Path_curvature : Constant  Value=path_curvature
  Scaling factor : Gain  Gain=1/1000
  Scalling factor : Gain  Gain=1/1000
  Throttle Saturation : Saturate  UpperLimit=1  LowerLimit=-1
  advancedPID_speed_and_brake_control : MATLAB Function  TreatAsAtomicUnit=on
  calculate_path_curvature : MATLAB Function  TreatAsAtomicUnit=on
  Throttle : Outport
  Brake_command : Outport  Port=2
  path_curvature : Outport  Port=3
  min_safe_speed : Outport  Port=4
  wires:
  advancedPID_speed_and_brake_control/1(throttle) -> Scaling factor/1  "throttle"
  path/1 -> calculate_path_curvature/1(path)
  speed_act/1 -> advancedPID_speed_and_brake_control/3(speed_act)
  calculate_path_curvature/2(min_safe_speed) -> min_safe_speed/1, advancedPID_speed_and_brake_control/2(min_s_speed)  "min_s_speed"
  velocity_y/1 -> calculate_path_curvature/2(velocity_y)
  velocity_x/1 -> calculate_path_curvature/3(velocity_x)
  steering/1 -> calculate_path_curvature/4(steering_angel)
  calculate_path_curvature/1(path_curvature) -> path_curvature/1
  Constant3/1 -> advancedPID_speed_and_brake_control/7(Kp_speed)
  Path_curvature/1 -> advancedPID_speed_and_brake_control/1(path_curv)
  desired_speed/1 -> advancedPID_speed_and_brake_control/4(desired_speed)
  Constant2/1 -> advancedPID_speed_and_brake_control/6(Ki_speed)
  Constant1/1 -> advancedPID_speed_and_brake_control/5(Kd_speed)
  advancedPID_speed_and_brake_control/2(brake_cmd) -> Scalling factor/1  "Brake cmd"
  Scaling factor/1 -> Throttle Saturation/1
  Throttle Saturation/1 -> Throttle/1  "Throttle_command"
  Scalling factor/1 -> Brake Saturation/1
  Brake Saturation/1 -> Brake_command/1  "Brake_command"

== system Generic_13/CreateBus VhclCtrl/Stanley  steering & speed//Brake controller/Stanley_controller_with_thottle_and_brake_commands/Stanley steering + PID speed controller/Subsystem1 ==
  desired_speed : Inport
  curvature : Inport  Port=2
  min_safe_speed : Inport  Port=3
  2-D Lookup Table : Lookup_n-D  BreakpointsForDimension1=speed  BreakpointsForDimension2=curvature  Table=brake_select  InternalRulePriority=Speed  RndMeth=Simplest
      settings: InputPortMap=u0,u1
  Divide : Product  Inputs=*/
  MATLAB Function : MATLAB Function  Commented=on  TreatAsAtomicUnit=on
  Read CM Dict : CarMaker4SL/Read CM Dict  xname=Sensor.Road.VehSensor_0.Path.CurveXY  xsync=off  xstime=Continuous
  Scope2 : Scope
  Target_speed : Outport
  curv : Outport  Port=2
  speed : Outport  Port=3
  wires:
  Divide/1 -> speed/1, Target_speed/1, Scope2/1
  2-D Lookup Table/1 -> Divide/2
  desired_speed/1 -> 2-D Lookup Table/1, Divide/1
  min_safe_speed/1 -> MATLAB Function/2(min_safe_speed)
  curvature/1 -> MATLAB Function/1(u)
  Read CM Dict/1 -> curv/1, 2-D Lookup Table/2

== system Generic_13/CreateBus VhclCtrl/Stanley  steering & speed//Brake controller/Road sensor set & path planning/Road sensor set & path planning/A* star path planning/Signal_smoothing ==
  Signal_In : Inport
  Smoothing1 : Subsystem
  Smoothing2 : Subsystem
  Smoothing4 : Subsystem
  smoothed_width : Outport
  wires:
  Signal_In/1 -> Smoothing1/1(Signal_In)
  Smoothing1/1(Signal_Out) -> Smoothing2/1(Signal_In)  "steering_signal"
  Smoothing2/1(Signal_Out) -> Smoothing4/1(Signal_In)  "steering_signal"
  Smoothing4/1(Signal_Out) -> smoothed_width/1  "smoothed_width"

== system Generic_13/CreateBus VhclCtrl/Stanley  steering & speed//Brake controller/Road sensor set & path planning/Road sensor set & path planning/A* star path planning/Smoothing3 ==
  Signal_In : Inport
  Add : Sum  Inputs=++++
  Delay : Delay  InitialCondition=0.1
  Delay1 : Delay  DelayLength=4  InitialCondition=0.1
  Delay2 : Delay  DelayLength=5  InitialCondition=0.1
  Gain : Gain  Gain=0.35
  Gain1 : Gain  Gain=0.25
  Gain2 : Gain  Gain=0.25
  Gain3 : Gain  Gain=0.15
  Signal_Out : Outport  VectorParamsAs1DForOutWhenUnconnected=off
  wires:
  Gain3/1 -> Add/4
  Delay2/1 -> Gain3/1
  Gain2/1 -> Add/3
  Add/1 -> Signal_Out/1, Delay/1, Delay1/1, Delay2/1
  Delay1/1 -> Gain2/1
  Gain/1 -> Add/1
  Delay/1 -> Gain1/1
  Signal_In/1 -> Gain/1
  Gain1/1 -> Add/2

== system Generic_13/CreateBus VhclCtrl/Stanley  steering & speed//Brake controller/Road sensor set & path planning/Road sensor set & path planning/Be'zeir path planning/Signal_smoothing ==
  Signal_In : Inport
  Smoothing1 : Subsystem
  Smoothing2 : Subsystem
  Smoothing4 : Subsystem
  smoothed_width : Outport
  wires:
  Smoothing4/1(Signal_Out) -> smoothed_width/1  "smoothed_width"
  Smoothing2/1(Signal_Out) -> Smoothing4/1(Signal_In)  "steering_signal"
  Smoothing1/1(Signal_Out) -> Smoothing2/1(Signal_In)  "steering_signal"
  Signal_In/1 -> Smoothing1/1(Signal_In)

== system Generic_13/CreateBus VhclCtrl/Stanley  steering & speed//Brake controller/Road sensor set & path planning/Road sensor set & path planning/Be'zeir path planning/Smoothing3 ==
  Signal_In : Inport
  Add : Sum  Inputs=++++
  Delay : Delay  InitialCondition=0.1
  Delay1 : Delay  DelayLength=4  InitialCondition=0.1
  Delay2 : Delay  DelayLength=5  InitialCondition=0.1
  Gain : Gain  Gain=0.35
  Gain1 : Gain  Gain=0.25
  Gain2 : Gain  Gain=0.25
  Gain3 : Gain  Gain=0.15
  Signal_Out : Outport  VectorParamsAs1DForOutWhenUnconnected=off
  wires:
  Gain1/1 -> Add/2
  Signal_In/1 -> Gain/1
  Delay/1 -> Gain1/1
  Gain/1 -> Add/1
  Delay1/1 -> Gain2/1
  Add/1 -> Delay2/1, Delay1/1, Delay/1, Signal_Out/1
  Gain2/1 -> Add/3
  Delay2/1 -> Gain3/1
  Gain3/1 -> Add/4

== system Generic_13/CreateBus VhclCtrl/Stanley  steering & speed//Brake controller/Road sensor set & path planning/Road sensor set & path planning/Car_yaw_rate/ Path_expanding1 ==
  X-path : Inport
  Y_path : Inport  Port=2
  Delay10 : Delay  DelayLength=6
  Delay11 : Delay  DelayLength=8
  Delay37 : Delay
  Delay38 : Delay  DelayLength=4
  Delay4 : Delay
  Delay5 : Delay  DelayLength=6
  Delay6 : Delay  DelayLength=8
  Delay9 : Delay  DelayLength=4
  Mux1 : Mux  Inputs=5
  Mux2 : Mux  Inputs=5
  Reshape1 : Reshape  OutputDimensionality=Customize  OutputDimensions=[1,5]
  Reshape2 : Reshape  OutputDimensionality=Customize  OutputDimensions=[1,5]
  x_path : Outport
  y_path : Outport  Port=2
  wires:
  Mux2/1 -> Reshape2/1
  Reshape2/1 -> x_path/1
  Delay11/1 -> Mux1/5
  Delay10/1 -> Mux1/4
  Delay9/1 -> Mux1/3
  Delay4/1 -> Mux1/2
  Reshape1/1 -> y_path/1
  Mux1/1 -> Reshape1/1
  Delay38/1 -> Mux2/3
  Delay6/1 -> Mux2/5
  Delay37/1 -> Mux2/2
  Delay5/1 -> Mux2/4
  Y_path/1 -> Delay11/1, Delay10/1, Delay9/1, Delay4/1, Mux1/1
  X-path/1 -> Delay6/1, Delay5/1, Delay37/1, Delay38/1, Mux2/1
